simulink model "task6"  (R2025b)
settings: Solver=VariableStepAuto  StartTime=0.0  StopTime=24  RelTol=1e-3
values from neighbouring files (symbols this model uses):
  Ad = sys_d.A    [task5_6.m]
  Bd = Bd_ext(:, 1:3)    [task5_6.m]
  Cd = sys_d.C    [task5_6.m]
  Dd = Dd_ext(:, 1:3)    [task5_6.m]
  Ed = Bd_ext(:, 4:5)    [task5_6.m]
  Pf = 1.5    [init.m]
  Pr = 7.0    (= 7)    [init.m]
  Qp_eq = 500    [task5_6.m]
  Sb_eq = 0.60    (= 0.6)    [task5_6.m]
  Ta_eq = 5    [task5_6.m]
  Te_eq = 24    [task5_6.m]
  Tp_eq = 5    [task5_6.m]
  Ts = 0.1    [init.m]    (also in run_task7.m = Ts_vec(k))
  ub_eq = 0.0    (= 0)    [task5_6.m]
  uf_eq = 0.5    [task5_6.m]
  ur_eq = (ke*(Te_eq - Ta_eq) + Qp_eq) / kr    [task5_6.m]
libraries: slpidlib x2
settings Model: Creator=davide  LastModifiedBy=davide

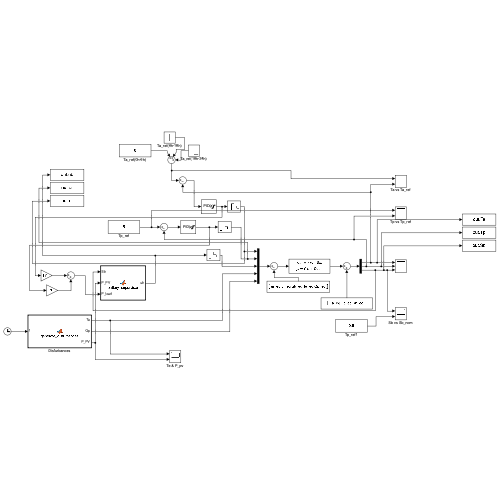
[thumbnail: Simulink's stored preview of the top-level diagram]
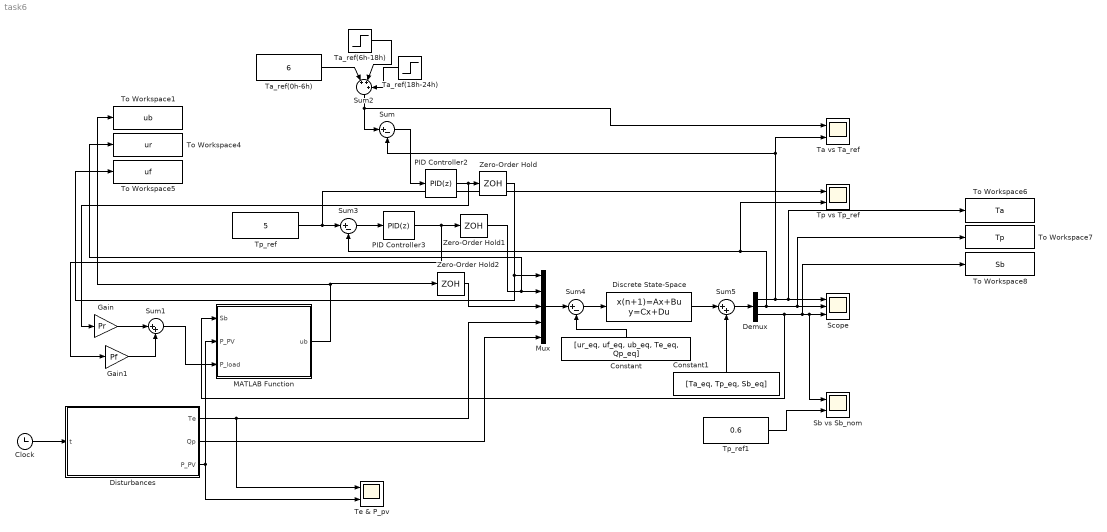
== system task6 ==
  Clock : Clock
  Constant : Constant  Value=[ur_eq, uf_eq, ub_eq, Te_eq, Qp_eq]
  Constant1 : Constant  Value=[Ta_eq, Tp_eq, Sb_eq]
  Demux : Demux  Outputs=3
  Discrete State-Space : DiscreteStateSpace  A=Ad  B=[Bd, Ed]  C=Cd  D=[Dd, zeros(3,2)]  InitialCondition=[10-5; 11.5-5; 0.55-0.60]  SampleTime=Ts
  Disturbances : MATLAB Function  TreatAsAtomicUnit=on
  Gain : Gain  Gain=Pr
  Gain1 : Gain  Gain=Pf
  MATLAB Function : MATLAB Function  TreatAsAtomicUnit=on
  Mux : Mux  Inputs=5
  PID Controller2 : slpidlib/PID Controller  Controller=PID  Form=Parallel  TimeDomain=Discrete-time  UseExternalTs=off  SampleTime=Ts  IntegratorMethod=Forward Euler  FilterMethod=Forward Euler  ControllerParametersSource=internal  P=-0.05  I=-0.025  UseKiTs=off  D=0  UseExternalDerivativeSource=off  N=100  UseFilter=on  TunerSelectOption=Transfer Function Based (PID Tuner App)  InitialConditionSource=internal  InitialConditionForIntegrator=0  InitialConditionForFilter=0  DifferentiatorICPrevScaledInput=0  ExternalReset=none  TrackingMode=off  Kt=1  LimitOutput=on  SatLimitsSource=internal  UpperSaturationLimit=1  LowerSaturationLimit=0  LinearizeAsGain=on  AntiWindupMode=back-calculation  Kb=1  LimitIntegrator=off  UpperIntegratorSaturationLimit=inf  LowerIntegratorSaturationLimit=-inf  POutMin=[]  POutMax=[]  IOutMin=[]  IOutMax=[]  DOutMin=[]  DOutMax=[]  NOutMin=[]  NOutMax=[]  SumOutMin=[]  SumOutMax=[]  SaturationOutMin=[]  SaturationOutMax=[]  PParamMin=[]  PParamMax=[]  IParamMin=[]  IParamMax=[]  DParamMin=[]  DParamMax=[]  NParamMin=[]  NParamMax=[]  KbParamMin=[]  KbParamMax=[]  KtParamMin=[]  KtParamMax=[]  KbOutMin=[]  KbOutMax=[]  KtOutMin=[]  KtOutMax=[]  IntegratorOutMin=[]  IntegratorOutMax=[]  FilterOutMin=[]  FilterOutMax=[]  SumI1OutMin=[]  SumI1OutMax=[]  SumI2OutMin=[]  SumI2OutMax=[]  SumI3OutMin=[]  SumI3OutMax=[]  SumI4OutMin=[]  SumI4OutMax=[]  SumDOutMin=[]  SumDOutMax=[]  DifferentiatorOutMin=[]  DifferentiatorOutMax=[]  FilterDiffOutCoefMin=[]  FilterDiffOutCoefMax=[]  ReciprocalOutMin=[]  ReciprocalOutMax=[]  SumDenOutMin=[]  SumDenOutMax=[]  SumNumOutMin=[]  SumNumOutMax=[]  DivideOutMin=[]  DivideOutMax=[]  UdiffTsProdOutMin=[]  UdiffTsProdOutMax=[]  NTsProdOutMin=[]  NTsProdOutMax=[]  UintegralTsProdOutMin=[]  UintegralTsProdOutMax=[]  UngainTsProdOutMin=[]  UngainTsProdOutMax=[]  ClampingZeroOutDataTypeStr=Inherit: Inherit via back propagation  ClampingZeroOutMin=[]  ClampingZeroOutMax=[]  FilterDenConstantOutDataTypeStr=Inherit: Inherit via back propagation  FilterDenConstantOutMin=[]  FilterDenConstantOutMax=[]  PCopyOutDataTypeStr=Inherit: Inherit via back propagation  PCopyOutMin=[]  PCopyOutMax=[]  NCopyOutDataTypeStr=Inherit: Inherit via back propagation  NCopyOutMin=[]  NCopyOutMax=[]  IntegratorContinuousStateAttributes=''  IntegratorStateMustResolveToSignalObject=off  IntegratorRTWStateStorageClass=Auto  FilterContinuousStateAttributes=''  FilterStateMustResolveToSignalObject=off  FilterRTWStateStorageClass=Auto  ParallelPVariant=InternalParameters  IdealPVariant=Disabled  IVariant=InternalParameters  DVariant=InternalParameters  IntegratorVariant=Discrete  SatVariant=Enabled  AWVariant=BackCalculation  PCopyVariant=Disabled  TRVariant=Disabled  FdbkBlocksVariant=Forward  IdealPFdbkVariant=Disabled  SatFdbkVariant=Disabled  DerivativeFilterVariant=ForwardEulerFilter  NVariant=InternalParameters  NCopyVariant=Disabled  FilterICVariant=InternalICsFilter  IntegratorICVariant=InternalICs  ExternalResetVariant=Disabled  TRSumVariant=Passthrough  SumFdbkVariant=Disabled  SumVariant=Sum_PID  TsampFilterVariant=InternalTs  TsampNgainVariant=Passthrough  TsampIntegralVariant=Disabled_SignalSpec  ExternalSaturationOutDataTypeStr=Inherit: Same as second input  DerivativeSourceVariant=ErrorSignal  PreIntVariant=InternalPreInt
  PID Controller3 : slpidlib/PID Controller  Controller=PID  Form=Parallel  TimeDomain=Discrete-time  UseExternalTs=off  SampleTime=Ts  IntegratorMethod=Forward Euler  FilterMethod=Forward Euler  ControllerParametersSource=internal  P=-0.05  I=-0.025  UseKiTs=off  D=0  UseExternalDerivativeSource=off  N=100  UseFilter=on  TunerSelectOption=Transfer Function Based (PID Tuner App)  InitialConditionSource=internal  InitialConditionForIntegrator=0  InitialConditionForFilter=0  DifferentiatorICPrevScaledInput=0  ExternalReset=none  TrackingMode=off  Kt=1  LimitOutput=on  SatLimitsSource=internal  UpperSaturationLimit=1  LowerSaturationLimit=0  LinearizeAsGain=on  AntiWindupMode=back-calculation  Kb=1  LimitIntegrator=off  UpperIntegratorSaturationLimit=inf  LowerIntegratorSaturationLimit=-inf  POutMin=[]  POutMax=[]  IOutMin=[]  IOutMax=[]  DOutMin=[]  DOutMax=[]  NOutMin=[]  NOutMax=[]  SumOutMin=[]  SumOutMax=[]  SaturationOutMin=[]  SaturationOutMax=[]  PParamMin=[]  PParamMax=[]  IParamMin=[]  IParamMax=[]  DParamMin=[]  DParamMax=[]  NParamMin=[]  NParamMax=[]  KbParamMin=[]  KbParamMax=[]  KtParamMin=[]  KtParamMax=[]  KbOutMin=[]  KbOutMax=[]  KtOutMin=[]  KtOutMax=[]  IntegratorOutMin=[]  IntegratorOutMax=[]  FilterOutMin=[]  FilterOutMax=[]  SumI1OutMin=[]  SumI1OutMax=[]  SumI2OutMin=[]  SumI2OutMax=[]  SumI3OutMin=[]  SumI3OutMax=[]  SumI4OutMin=[]  SumI4OutMax=[]  SumDOutMin=[]  SumDOutMax=[]  DifferentiatorOutMin=[]  DifferentiatorOutMax=[]  FilterDiffOutCoefMin=[]  FilterDiffOutCoefMax=[]  ReciprocalOutMin=[]  ReciprocalOutMax=[]  SumDenOutMin=[]  SumDenOutMax=[]  SumNumOutMin=[]  SumNumOutMax=[]  DivideOutMin=[]  DivideOutMax=[]  UdiffTsProdOutMin=[]  UdiffTsProdOutMax=[]  NTsProdOutMin=[]  NTsProdOutMax=[]  UintegralTsProdOutMin=[]  UintegralTsProdOutMax=[]  UngainTsProdOutMin=[]  UngainTsProdOutMax=[]  ClampingZeroOutDataTypeStr=Inherit: Inherit via back propagation  ClampingZeroOutMin=[]  ClampingZeroOutMax=[]  FilterDenConstantOutDataTypeStr=Inherit: Inherit via back propagation  FilterDenConstantOutMin=[]  FilterDenConstantOutMax=[]  PCopyOutDataTypeStr=Inherit: Inherit via back propagation  PCopyOutMin=[]  PCopyOutMax=[]  NCopyOutDataTypeStr=Inherit: Inherit via back propagation  NCopyOutMin=[]  NCopyOutMax=[]  IntegratorContinuousStateAttributes=''  IntegratorStateMustResolveToSignalObject=off  IntegratorRTWStateStorageClass=Auto  FilterContinuousStateAttributes=''  FilterStateMustResolveToSignalObject=off  FilterRTWStateStorageClass=Auto  ParallelPVariant=InternalParameters  IdealPVariant=Disabled  IVariant=InternalParameters  DVariant=InternalParameters  IntegratorVariant=Discrete  SatVariant=Enabled  AWVariant=BackCalculation  PCopyVariant=Disabled  TRVariant=Disabled  FdbkBlocksVariant=Forward  IdealPFdbkVariant=Disabled  SatFdbkVariant=Disabled  DerivativeFilterVariant=ForwardEulerFilter  NVariant=InternalParameters  NCopyVariant=Disabled  FilterICVariant=InternalICsFilter  IntegratorICVariant=InternalICs  ExternalResetVariant=Disabled  TRSumVariant=Passthrough  SumFdbkVariant=Disabled  SumVariant=Sum_PID  TsampFilterVariant=InternalTs  TsampNgainVariant=Passthrough  TsampIntegralVariant=Disabled_SignalSpec  ExternalSaturationOutDataTypeStr=Inherit: Same as second input  DerivativeSourceVariant=ErrorSignal  PreIntVariant=InternalPreInt
  Sb vs Sb_nom : Scope  NumInputPorts=2
      settings: ActiveDisplayYMinimum=-1  ActiveDisplayYMaximum=1  DataLoggingVariableName=ScopeData3
  Scope : Scope  NumInputPorts=3
      settings: ActiveDisplayYMinimum=-0.81874999999999976  ActiveDisplayYMaximum=12.86875
  Sum : Sum  Inputs=|+-
  Sum1 : Sum  Inputs=|++
  Sum2 : Sum  Inputs=|+++
  Sum3 : Sum  Inputs=|+-
  Sum4 : Sum  Inputs=|+-
  Sum5 : Sum  Inputs=|++
  Ta vs Ta_ref : Scope  NumInputPorts=2
      settings: ActiveDisplayYMinimum=-1  ActiveDisplayYMaximum=1
  Ta_ref(0h-6h) : Constant  Value=6
  Ta_ref(18h-24h) : Step  Time=18  After=-1  SampleTime=0
  Ta_ref(6h-18h) : Step  Time=6  After=-1  SampleTime=0
  Te & P_pv : Scope  NumInputPorts=2
      settings: ActiveDisplayYMinimum=-3.9999999999999991  ActiveDisplayYMaximum=36  DataLoggingVariableName=ScopeData4
  To Workspace1 : ToWorkspace  VariableName=ub  SaveFormat=Timeseries  SampleTime=-1
      settings: Save2DSignal=2-D array (concatenate along first dimension)
  To Workspace4 : ToWorkspace  VariableName=ur  SaveFormat=Timeseries  SampleTime=-1
      settings: Save2DSignal=2-D array (concatenate along first dimension)
  To Workspace5 : ToWorkspace  VariableName=uf  SaveFormat=Timeseries  SampleTime=-1
      settings: Save2DSignal=2-D array (concatenate along first dimension)
  To Workspace6 : ToWorkspace  VariableName=Ta  SaveFormat=Timeseries  SampleTime=-1
      settings: Save2DSignal=2-D array (concatenate along first dimension)
  To Workspace7 : ToWorkspace  VariableName=Tp  SaveFormat=Timeseries  SampleTime=-1
      settings: Save2DSignal=2-D array (concatenate along first dimension)
  To Workspace8 : ToWorkspace  VariableName=Sb  SaveFormat=Timeseries  SampleTime=-1
      settings: Save2DSignal=2-D array (concatenate along first dimension)
  Tp vs Tp_ref : Scope  NumInputPorts=2
      settings: ActiveDisplayYMinimum=1.7593702953147823  ActiveDisplayYMaximum=12.582292189409468  DataLoggingVariableName=ScopeData2
  Tp_ref : Constant  Value=5
  Tp_ref1 : Constant  Value=0.6
  Zero-Order Hold : ZeroOrderHold  SampleTime=Ts
  Zero-Order Hold1 : ZeroOrderHold  SampleTime=Ts
  Zero-Order Hold2 : ZeroOrderHold  SampleTime=Ts
  wires:
  Clock/1 -> Disturbances/1(t)
  Ta_ref(18h-24h)/1 -> Sum2/3
  Ta_ref(6h-18h)/1 -> Sum2/2
  Ta_ref(0h-6h)/1 -> Sum2/1
  Sum/1 -> PID Controller2/1
  PID Controller2/1 -> Gain/1, Zero-Order Hold/1
  Tp_ref/1 -> Tp vs Tp_ref/1, Sum3/1
  Sum3/1 -> PID Controller3/1
  MATLAB Function/1(ub) -> To Workspace1/1, Zero-Order Hold2/1
  Disturbances/3(P_PV) -> MATLAB Function/2(P_PV), Te & P_pv/2
  Gain1/1 -> Sum1/2
  Gain/1 -> Sum1/1
  Sum1/1 -> MATLAB Function/3(P_load)
  Zero-Order Hold/1 -> To Workspace5/1, Mux/1
  PID Controller3/1 -> Gain1/1, Zero-Order Hold1/1
  Zero-Order Hold1/1 -> To Workspace4/1, Mux/2
  Zero-Order Hold2/1 -> Mux/3
  Disturbances/1(Te) -> Te & P_pv/1, Mux/4
  Disturbances/2(Qp) -> Mux/5
  Constant/1 -> Sum4/2
  Mux/1 -> Sum4/1
  Sum4/1 -> Discrete State-Space/1
  Discrete State-Space/1 -> Sum5/1
  Constant1/1 -> Sum5/2
  Sum5/1 -> Demux/1
  Demux/1 -> Scope/1, To Workspace6/1, Ta vs Ta_ref/2, Sum/2
  Demux/2 -> To Workspace7/1, Scope/2, Tp vs Tp_ref/2, Sum3/2
  Demux/3 -> To Workspace8/1, Sb vs Sb_nom/1, Scope/3, MATLAB Function/1(Sb)
  Sum2/1 -> Ta vs Ta_ref/1, Sum/1
  Tp_ref1/1 -> Sb vs Sb_nom/2

== matlab function task6/MATLAB Function ==
  data: Sb input; ub output; P_PV input; P_load input
function ub = battery_supervisor(Sb, P_PV, P_load)
    Sb_nom = 0.60;
    ub_max = 4.0;  % [kW] 
    ub_min = -4.0; % [kW] 
    
    % Calcolo del bilancio netto di potenza
    P_net = P_load - P_PV; 
    
    Kb = 100;

    % Se Sb < Sb_nom, P_soc diventa negativo (richiesta di ricarica)
    P_soc = -Kb * (Sb_nom - Sb); 
    
    % Azione richiesta teorica (Feedforward + Proporzionale)
    ub_req = P_net + P_soc;
    
    
    % Vincolo Bonus: "Battery charging only when surplus PV is available"
    % MASSIMIZZARE la sostenibilità
    if ub_req < 0 
        if P_net >= 0
            % Controlliamo il bilancio energetico reale. Se P_net è positivo, significa che i
            % motori stanno consumando più di quanto il sole produca. In questa situazione, 
            % non c'è energia solare in avanzo. Se caricassimo la batteria, staremmo letteralmente comprando energia dalla rete 
            % per metterla nella batteria, il che è uno spreco economico! Quindi blocchiamo la carica: ub_req = 0
            ub_req = 0;
        else
            % Surplus disponibile: carica la batteria ma senza superare il surplus stesso
            ub_req = max(ub_req, P_net); 
        end
    end
    
    % Limiti di sicurezza dello Stato di Carica (evitiamo i limiti fisici 0.15 e 0.95)
    if Sb <= 0.20 && ub_req > 0
        % Batteria prossima alla scarica critica: ferma l'erogazione
        ub_req = 0; 
    elseif Sb >= 0.90 && ub_req < 0
        % Batteria quasi piena: ferma la ricarica
        ub_req = 0; 
    end
    
    % Saturazione hardware dell'inverter (-4 <= ub <= 4 kW)
    ub = max(ub_min, min(ub_max, ub_req));
end

== matlab function task6/Disturbances ==
  data: t input; Te output; Qp output; P_PV output
function [Te, Qp, P_PV] = generate_disturbances(t)
    Rmax = 850; Pmax = 9.0;
    
    Te = 24 + 8 * sin(pi/12 * (t - 8));
    
    if t >= 6 && t <= 18
        Rs = Rmax * sin(pi * (t - 6) / 12);
    else
        Rs = 0;
    end
    P_PV = Pmax * (Rs / Rmax);
    
    % Thermal Charge   
    if t < 4
        Qp = 1200;
    elseif t < 10
        Qp = 600;
    else
        Qp = 250;
    end
end
